simulink model "PID_PalmSat"  (R2017b)
settings: Solver=VariableStepAuto  StartTime=0.0  StopTime=45  RelTol=1e-3
values from neighbouring files (symbols this model uses):
  B = ModeloSatelite.B    [PalmSatModelScript.m]
  Kt = Kw/0.00684    (= 25.0525729951)    [PalmSatModelScript.m]
  Kw = 60*2*pi/2200    (= 0.171359599287)    [PalmSatModelScript.m]
  La = 74.4*10^-6    (= 7.44e-05)    [PalmSatModelScript.m]
  Ra = 0.225    [PalmSatModelScript.m]
undefined symbols (not defined in the file or in its folder): IA, IB, IC, J, Kpx, Kpy, Kpz, Tdx, Tdy, Tdz, Tix, Tiy, Tiz
settings Model: Creator=Gpiaia  LastModifiedBy=Gpiaia

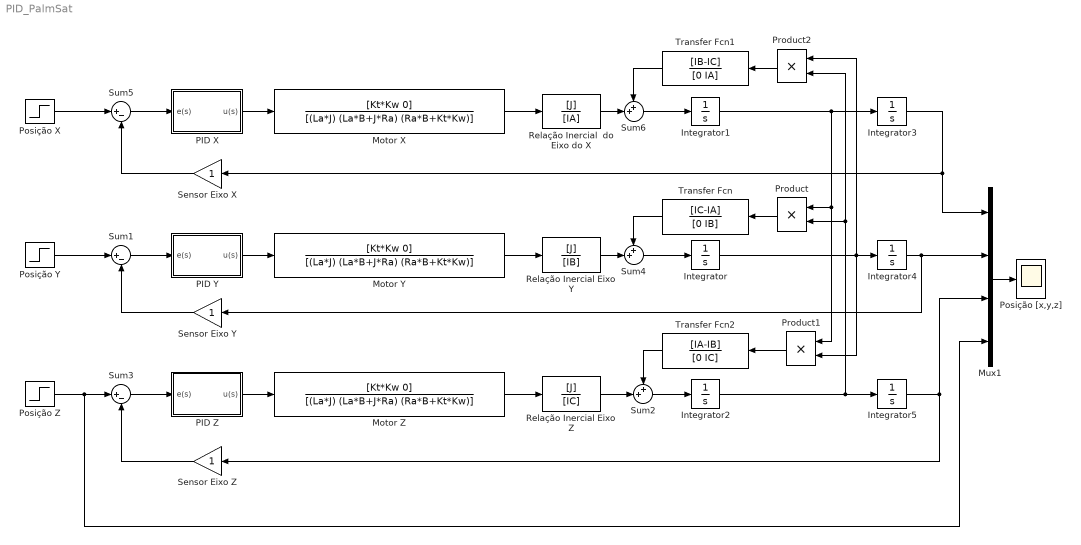
== system PID_PalmSat ==
  " Motor X" : TransferFcn  Numerator=[Kt*Kw 0]  Denominator=[(La*J) (La*B+J*Ra) (Ra*B+Kt*Kw)]
  Integrator{,1..5} (6 alike) : Integrator
  Motor Y : TransferFcn  Numerator=[Kt*Kw 0]  Denominator=[(La*J) (La*B+J*Ra) (Ra*B+Kt*Kw)]
  Motor Z : TransferFcn  Numerator=[Kt*Kw 0]  Denominator=[(La*J) (La*B+J*Ra) (Ra*B+Kt*Kw)]
  Mux1 : Mux
  PID X : Subsystem
  PID Y : Subsystem
  PID Z : Subsystem
  Posição [x,y,z] : Scope
  Posição X : Step  Time=5  After=0  SampleTime=0
  Posição Y : Step  Time=4  After=0  SampleTime=0
  Posição Z : Step  After=45  SampleTime=0
  Product : Product
  Product1 : Product
  Product2 : Product
  Relação Inercial Eixo Y : TransferFcn  Numerator=[J]  Denominator=[IB]
  Relação Inercial Eixo Z : TransferFcn  Numerator=[J]  Denominator=[IC]
  Relação Inercial  do Eixo do X : TransferFcn  Numerator=[J]  Denominator=[IA]
  Sensor Eixo X : Gain
  Sensor Eixo Y : Gain
  Sensor Eixo Z : Gain
  Sum1 : Sum  Inputs=|+-
  Sum2 : Sum  Inputs=++|
  Sum3 : Sum  Inputs=|+-
  Sum4 : Sum  Inputs=++|
  Sum5 : Sum  Inputs=|+-
  Sum6 : Sum  Inputs=++|
  Transfer Fcn : TransferFcn  Numerator=[IC-IA]  Denominator=[0 IB]
  Transfer Fcn1 : TransferFcn  Numerator=[IB-IC]  Denominator=[0 IA]
  Transfer Fcn2 : TransferFcn  Numerator=[IA-IB]  Denominator=[0 IC]
  wires:
  Relação Inercial Eixo Y/1 -> Sum4/2
  Relação Inercial Eixo Z/1 -> Sum2/2
  Posição X/1 -> Sum5/1
  Transfer Fcn/1 -> Sum4/1
  Mux1/1 -> Posição [x,y,z]/1
  Transfer Fcn2/1 -> Sum2/1
  Sensor Eixo Z/1 -> Sum3/2
  Transfer Fcn1/1 -> Sum6/1
  Relação Inercial  do Eixo do X/1 -> Sum6/2
  Sum4/1 -> Integrator/1
  Sensor Eixo X/1 -> Sum5/2
  Product1/1 -> Transfer Fcn2/1
  Integrator1/1 -> Integrator3/1, Product1/1, Product/1
  Motor Z/1 -> Relação Inercial Eixo Z/1
  Integrator/1 -> Product1/2, Product2/1, Integrator4/1
  Motor Y/1 -> Relação Inercial Eixo Y/1
  Integrator5/1 -> Mux1/3, Sensor Eixo Z/1
  Product2/1 -> Transfer Fcn1/1
  Posição Y/1 -> Sum1/1
  Sensor Eixo Y/1 -> Sum1/2
  Integrator3/1 -> Sensor Eixo X/1, Mux1/1
  Integrator2/1 -> Integrator5/1, Product2/2, Product/2
  " Motor X"/1 -> Relação Inercial  do Eixo do X/1
  Product/1 -> Transfer Fcn/1
  Sum6/1 -> Integrator1/1
  Integrator4/1 -> Sensor Eixo Y/1, Mux1/2
  Posição Z/1 -> Mux1/4, Sum3/1
  Sum2/1 -> Integrator2/1
  Sum3/1 -> PID Z/1(e(s))
  PID Z/1(u(s)) -> Motor Z/1
  Sum1/1 -> PID Y/1(e(s))
  PID Y/1(u(s)) -> Motor Y/1
  Sum5/1 -> PID X/1(e(s))
  PID X/1(u(s)) -> " Motor X"/1

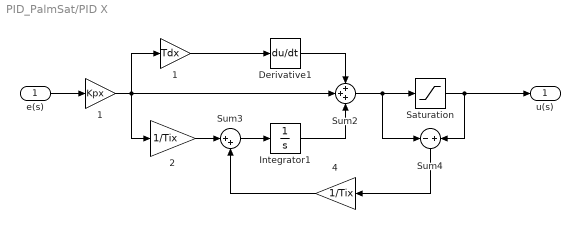
== system PID_PalmSat/PID X ==
  e(s) : Inport
  " 1" : Gain  Gain=Tdx
  "  2" : Gain  Gain=1/Tix
  "  4" : Gain  Gain=1/Tix
  " 1" : Gain  Gain=Kpx
  Derivative1 : Derivative
  Integrator1 : Integrator
  Saturation : Saturate  UpperLimit=5  LowerLimit=-5
  Sum2 : Sum  Inputs=+++
  Sum3 : Sum  Inputs=|++
  Sum4 : Sum  Inputs=-+
  u(s) : Outport
  wires:
  " 1"/1 -> Derivative1/1
  "  2"/1 -> Sum3/1
  "  4"/1 -> Sum3/2
  " 1"/1 -> " 1"/1, Sum2/2, "  2"/1
  Sum3/1 -> Integrator1/1
  Saturation/1 -> u(s)/1, Sum4/2
  Integrator1/1 -> Sum2/3
  Derivative1/1 -> Sum2/1
  Sum2/1 -> Sum4/1, Saturation/1
  Sum4/1 -> "  4"/1
  e(s)/1 -> " 1"/1

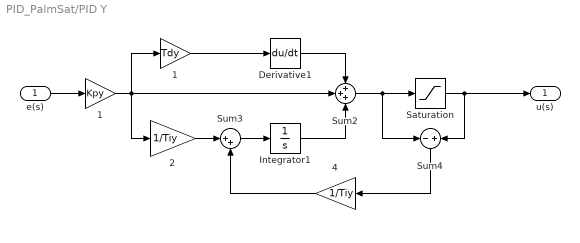
== system PID_PalmSat/PID Y ==
  e(s) : Inport
  " 1" : Gain  Gain=Tdy
  "  2" : Gain  Gain=1/Tiy
  "  4" : Gain  Gain=1/Tiy
  " 1" : Gain  Gain=Kpy
  Derivative1 : Derivative
  Integrator1 : Integrator
  Saturation : Saturate  UpperLimit=5  LowerLimit=-5
  Sum2 : Sum  Inputs=+++
  Sum3 : Sum  Inputs=|++
  Sum4 : Sum  Inputs=-+
  u(s) : Outport
  wires:
  " 1"/1 -> Derivative1/1
  "  2"/1 -> Sum3/1
  "  4"/1 -> Sum3/2
  " 1"/1 -> " 1"/1, Sum2/2, "  2"/1
  Sum3/1 -> Integrator1/1
  Saturation/1 -> u(s)/1, Sum4/2
  Integrator1/1 -> Sum2/3
  Derivative1/1 -> Sum2/1
  Sum2/1 -> Sum4/1, Saturation/1
  Sum4/1 -> "  4"/1
  e(s)/1 -> " 1"/1

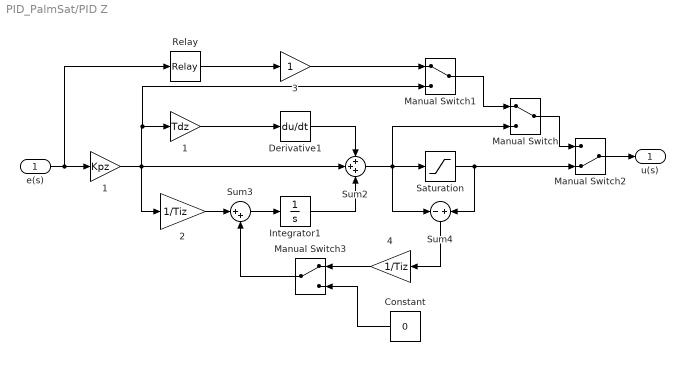
== system PID_PalmSat/PID Z ==
  e(s) : Inport
  " 1" : Gain  Gain=Tdz
  " 3" : Gain
  "  2" : Gain  Gain=1/Tiz
  "  4" : Gain  Gain=1/Tiz
  " 1" : Gain  Gain=Kpz
  Constant : Constant  Value=0
  Derivative1 : Derivative
  Integrator1 : Integrator
  Manual Switch : ManualSwitch
  Manual Switch1 : ManualSwitch
  Manual Switch2 : ManualSwitch  CurrentSetting=0
  Manual Switch3 : ManualSwitch
  Relay : Relay  OnSwitchValue=+0.01  OffSwitchValue=-0.01  OnOutputValue=+1  OffOutputValue=-1
  Saturation : Saturate  UpperLimit=200  LowerLimit=-200
  Sum2 : Sum  Inputs=+++
  Sum3 : Sum  Inputs=|++
  Sum4 : Sum  Inputs=-+
  u(s) : Outport
  wires:
  " 1"/1 -> Derivative1/1
  "  2"/1 -> Sum3/1
  " 1"/1 -> Manual Switch1/2, " 1"/1, Sum2/2, "  2"/1
  Sum3/1 -> Integrator1/1
  Saturation/1 -> Manual Switch2/2, Sum4/2
  Integrator1/1 -> Sum2/3
  Derivative1/1 -> Sum2/1
  Sum2/1 -> Saturation/1, Manual Switch/2, Sum4/1
  Sum4/1 -> "  4"/1
  e(s)/1 -> Relay/1, " 1"/1
  Relay/1 -> " 3"/1
  " 3"/1 -> Manual Switch1/1
  Manual Switch1/1 -> Manual Switch/1
  Manual Switch2/1 -> u(s)/1
  Manual Switch/1 -> Manual Switch2/1
  Manual Switch3/1 -> Sum3/2
  "  4"/1 -> Manual Switch3/1
  Constant/1 -> Manual Switch3/2
